simulink model "CBE_145_HW4_P3"  (R2020b)
settings: Solver=VariableStepAuto  StartTime=0.0  StopTime=50  RelTol=1e-3
settings Model: SimulationMode=accelerator  Creator=Jesus Vergara  LastModifiedBy=Jesus Vergara

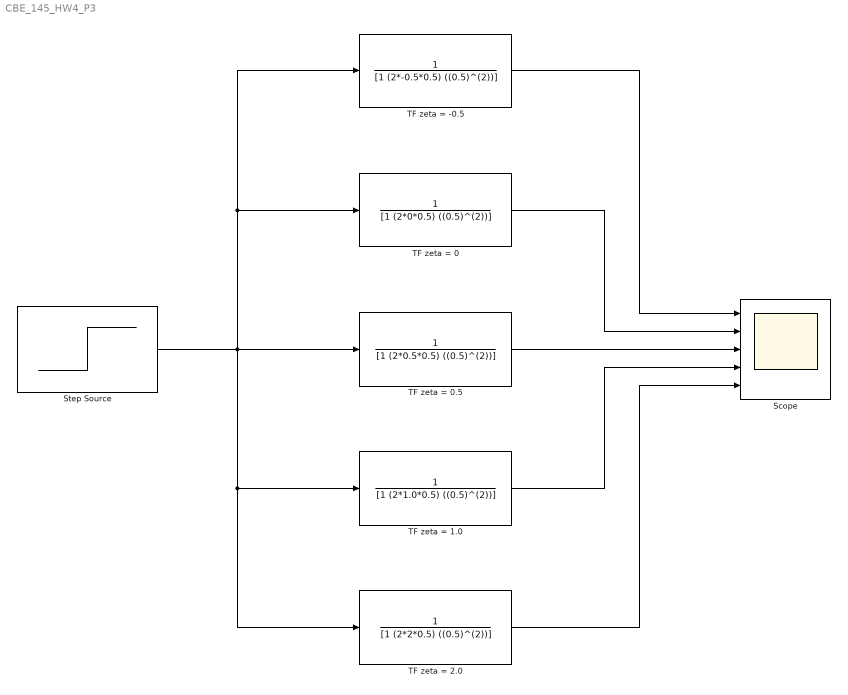
== system CBE_145_HW4_P3 ==
  Scope : Scope  NumInputPorts=5
  Step Source : Step  After=2  SampleTime=0
  TF zeta = -0.5 : TransferFcn  Denominator=[1 (2*-0.5*0.5) ((0.5)^(2))]
  TF zeta = 0 : TransferFcn  Denominator=[1 (2*0*0.5) ((0.5)^(2))]
  TF zeta = 0.5 : TransferFcn  Denominator=[1 (2*0.5*0.5) ((0.5)^(2))]
  TF zeta = 1.0 : TransferFcn  Denominator=[1 (2*1.0*0.5) ((0.5)^(2))]
  TF zeta = 2.0 : TransferFcn  Denominator=[1 (2*2*0.5) ((0.5)^(2))]
  wires:
  Step Source/1 -> TF zeta = 2.0/1, TF zeta = 1.0/1, TF zeta = 0.5/1, TF zeta = 0/1, TF zeta = -0.5/1
  TF zeta = -0.5/1 -> Scope/1
  TF zeta = 0/1 -> Scope/2
  TF zeta = 0.5/1 -> Scope/3
  TF zeta = 1.0/1 -> Scope/4
  TF zeta = 2.0/1 -> Scope/5
